simulink model "Nanogrid"  (R2026a)
settings: Solver=VariableStepAuto  StopTime=3
PreLoadFcn:
  | NanogridParam
undefined symbols (not defined in the file): baseLoad, bessSystem, bessVoltage, DiscIntNeverNeededParam, ee_sli_rtmsupport, gcbh, gflInverter, gfmInverter, nanoLoad, PV, PVInverter, ref, solar, solarInsolationChange, Ts
libraries: nesl_utility x51, eeGeneralControl x38, ee_lib x33, fl_lib x24, simulink x20, eeTransforms x13, slpidlib x8, nesl_utility_internal x4, sl_signal_attributes x4, sl_discontinuities x4, eeSinusoidalMeasurementV2 x3, batteryecm_lib x2
(part 3 of 6)

== system Nanogrid/BESS Integrated/Detailed/BESS Controller/Grid Forming ==
  VRef : Inport
  FRef : Inport  Port=2
  PRef : Inport  Port=3
  QRef : Inport  Port=4
  Mode : Inport  Port=5
  Reset : Inport  Port=6
  Bus Element In : Inport  Port=7  PortName=VIBus  Element=Vabc
  BusElementIn : Inport  Port=7  PortName=VIBus  Element=Iabc
  Current Limiting : Subsystem
  Grid Voltage Reactive Power Support : Subsystem
  Measurement : Subsystem
      mask Display: image('meas2_1_7_7_2.png');
  Power Control : Subsystem
  Subsystem2 : Subsystem
      settings: PortSchema="{\"entries\":[{\"content\":{\"sides\":[{\"content\":{\"connectorIds\":[\"Out1\"]},\"type\":\"ConnectorPlacement.EquallySpacedRectSide\",\"uuid\":\"7526c1f7-0aba-4355-8bbd-47d168879ecb\"},{\"content\":{\"connectorIds\":[\"In1\",\"In2\"],\"side\":\"RIGHT\"},\"type\":\"ConnectorPlacement.EquallySpacedRectSide\",\"uuid\":\"1dda9693-ec76-4df0-8ad4-aaa83d2574b3\"},{\"content\":{\"side\":\"TOP\"},\"type\":\"ConnectorPlacement.EquallySpacedRectSide\",\"uuid\":\"71ea411b-eb5f-4279-ae23-08ebb3ff1ed6\"}]},\"type\":\"ConnectorPlacement.EquallySpacedConnector\",\"uuid\":\"19864e0c-0998-460d-9705-13c69283d4ec\"}],\"packageUris\":[\"http://schema.mathworks.com/mf0/Connector/R2020b\"],\"version\":\"1.0\"}"
  Terminator : Terminator
  Terminator1 : Terminator
  Terminator2 : Terminator
  VoltageCurrentControl : Subsystem
      settings: PortSchema="{\"entries\":[{\"content\":{\"sides\":[{\"content\":{\"connectorIds\":[\"In1\",\"In2\",\"In3\"]},\"type\":\"ConnectorPlacement.EquallySpacedRectSide\",\"uuid\":\"0bf15a12-7bc0-47e4-89bd-435769673763\"},{\"content\":{\"connectorIds\":[\"Out1\"],\"side\":\"RIGHT\"},\"type\":\"ConnectorPlacement.EquallySpacedRectSide\",\"uuid\":\"44a15d74-8878-4ec6-abe4-be0b1b609519\"},{\"content\":{\"connectorIds\":[\"In4\"],\"side\":\"TOP\"},\"type\":\"ConnectorPlacement.EquallySpacedRectSide\",\"uuid\":\"7a96781e-5638-4b2a-8101-d5785aae9f0f\"}]},\"type\":\"ConnectorPlacement.EquallySpacedConnector\",\"uuid\":\"4b3373ad-cf20-4175-894e-3bd1604dd0ce\"}],\"packageUris\":[\"http://schema.mathworks.com/mf0/Connector/R2020b\"],\"version\":\"1.0\"}"
  mabc : Outport
  wires:
  Reset/1 -> Subsystem2/2(Reset), VoltageCurrentControl/3(Reset)
  Mode/1 -> Power Control/6(CntrlFlag)
  VRef/1 -> Power Control/4(Vref)
  FRef/1 -> Power Control/5(Fref)
  Measurement/4(fmeas) -> Terminator2/1
  Grid Voltage Reactive Power Support/2(Qref) -> Power Control/3(Qref)
  Grid Voltage Reactive Power Support/1(Pref) -> Power Control/2(Pref)
  PRef/1 -> Grid Voltage Reactive Power Support/2(PrefInput)
  QRef/1 -> Grid Voltage Reactive Power Support/3(QrefInput)
  Current Limiting/1(currentLimiting) -> VoltageCurrentControl/1(currentLimiting)
  Power Control/2(activeControl) -> VoltageCurrentControl/2(activeControl)
  Power Control/1(reactiveControl) -> Current Limiting/2(reactiveControl)
  Power Control/3(angle) -> Measurement/3(Angle)
  Measurement/1(measure) -> Grid Voltage Reactive Power Support/1(measure), Power Control/1(measure), VoltageCurrentControl/4(measure), Current Limiting/1(measure)
  Measurement/3(Qmeas) -> Terminator1/1
  Measurement/2(Pmeas) -> Terminator/1
  BusElementIn/1 -> Measurement/2(Igabc)
  Bus Element In/1 -> Measurement/1(Vgabcc)
  VoltageCurrentControl/1(mabc) -> Subsystem2/1(In)
  Subsystem2/1(mabc) -> mabc/1

== system Nanogrid/BESS Integrated/Detailed/BESS Plant/Converter ==
  mabc : Inport
  Average : Subsystem  VariantControl=Average
  Switching : Subsystem  VariantControl=Switching
  + : PMIOPort  Side=Left
  - : PMIOPort  Port=2  Side=Left
  ~ : PMIOPort  Port=3  Side=Right

== system Nanogrid/BESS Integrated/Detailed/Filter & Measurements/PLL & Measurements ==
  V : Inport
  I : Inport  Port=2
  Measurement1 : Subsystem
  Measurement2 : Subsystem
  Subsystem : Subsystem
  Out Bus Element : Outport  PortName=VIbus  Element=Vq
  Out Bus Element1 : Outport  PortName=VIbus  Element=Vd
  Out Bus Element2 : Outport  PortName=VIbus  Element=Freq
  Out Bus Element3 : Outport  PortName=VIbus  Element=Theta
  Out Bus Element4 : Outport  PortName=VIbus  Element=Vmag
  Out Bus Element5 : Outport  PortName=VIbus  Element=Iq
  Out Bus Element6 : Outport  PortName=VIbus  Element=Id
  Out Bus Element7 : Outport  PortName=VIbus  Element=Iabc
  Out Bus Element8 : Outport  PortName=VIbus  Element=Vabc
  wires:
  Subsystem/6(Id1) -> Out Bus Element6/1
  Subsystem/7(Iq1) -> Out Bus Element5/1
  Measurement1/1(Vg) -> Subsystem/2(Iabc), Out Bus Element7/1
  I/1 -> Measurement1/1(u)
  Subsystem/1(mag) -> Out Bus Element4/1
  Measurement2/1(Vg) -> Subsystem/1(Vabc), Out Bus Element8/1
  Subsystem/4(Vd) -> Out Bus Element1/1
  Subsystem/3(angle) -> Out Bus Element3/1
  Subsystem/5(Vq) -> Out Bus Element/1
  Subsystem/2(freq) -> Out Bus Element2/1
  V/1 -> Measurement2/1(u)

== system Nanogrid/BESS Integrated/Simplified/Grid Following/Measurements ==
  Current and Voltage Sensor (Three-Phase)5 : ee_lib/Sensors & Transducers/Current and Voltage Sensor (Three-Phase)  vMeasurementType=ee.enum.vmeasurement.lg  outputUnit=ee.enum.unit.pu  SRated=plantRating*1000 A*V  VRated=Vac V  I_specify=off  I_priority=None  I=[0, 0, 0] A  I_nominal_specify=off  I_nominal_value=1  I_nominal_unit=A  V_specify=off  V_priority=None  V=[0, 0, 0] V  V_nominal_specify=off  V_nominal_value=1  V_nominal_unit=V
      settings: InternalSimscapePortConfiguration="{\"Bottom\":[],\"Left\":[{\"id\":\"N1\",\"label\":\"~1\",\"type\":\"foundation.electrical.three_phase\"}],\"Right\":[{\"id\":\"V_output\",\"label\":\"V\",\"type\":\"output\"},{\"id\":\"I_output\",\"label\":\"I\",\"type\":\"output\"},{\"id\":\"N2\",\"label\":\"~2\",\"type\":\"foundation.electrical.three_phase\"}],\"Top\":[]}"
  Gain1 : Gain  Gain=1/(plantRating*1000)
  Gain2 : Gain  Gain=1/(plantRating*1000)
  Low-Pass Filter (Discrete or Continuous)1 : eeGeneralControl/Low-Pass Filter (Discrete or Continuous)  K=1  T=0.1  B=inf  A=-inf  init_option=Inherited from block input  x0=0  Ts=-1
  Low-Pass Filter (Discrete or Continuous)2 : eeGeneralControl/Low-Pass Filter (Discrete or Continuous)  K=1  T=0.1  B=inf  A=-inf  init_option=Inherited from block input  x0=0  Ts=-1
  PS-Simulink Converter{,1..3} (4 alike) : nesl_utility/PS-Simulink Converter  PhysicalDomain=network_engine_domain  SubClassName=ps_output  LeftPortType=input  RightPortType=output  PseudoPeriodic=off  Frequencies=[]  VectorFormat=inherit  Unit=inherit  AffineConversion=off
  Power Sensor (Three-Phase) : ee_lib/Sensors & Transducers/Power Sensor (Three-Phase)  load_type=ee.enum.passive.type_balanced.balanced  f0=60 Hz
      settings: InternalSimscapePortConfiguration="{\"Bottom\":[],\"Left\":[{\"id\":\"N1\",\"label\":\"~1\",\"type\":\"foundation.electrical.three_phase\"}],\"Right\":[{\"id\":\"N2\",\"label\":\"~2\",\"type\":\"foundation.electrical.three_phase\"}],\"Top\":[{\"id\":\"Pm\",\"label\":\"P\",\"type\":\"output\"},{\"id\":\"Qm\",\"label\":\"Q\",\"type\":\"output\"}]}"
  In : PMIOPort  Side=Left
  ~ : PMIOPort  Port=2  Side=Right
  P : Outport
  Q : Outport  Port=2
  V : Outport  Port=3
  I : Outport  Port=4
  wires:
  Gain2/1 -> Q/1
  Gain1/1 -> P/1
  PS-Simulink Converter3/1 -> I/1
  PS-Simulink Converter2/1 -> V/1
  Low-Pass Filter (Discrete or Continuous)2/1 -> Gain2/1
  Low-Pass Filter (Discrete or Continuous)1/1 -> Gain1/1
  PS-Simulink Converter1/1 -> Low-Pass Filter (Discrete or Continuous)2/1
  PS-Simulink Converter/1 -> Low-Pass Filter (Discrete or Continuous)1/1
  connections:
  PS-Simulink Converter3/LConn1 -- Current and Voltage Sensor (Three-Phase)5/RConn2
  Power Sensor (Three-Phase)/RConn1 -- Current and Voltage Sensor (Three-Phase)5/LConn1
  PS-Simulink Converter1/LConn1 -- Power Sensor (Three-Phase)/LConn3
  ~/RConn1 -- Current and Voltage Sensor (Three-Phase)5/RConn3
  In/RConn1 -- Power Sensor (Three-Phase)/LConn1
  PS-Simulink Converter/LConn1 -- Power Sensor (Three-Phase)/LConn2
  PS-Simulink Converter2/LConn1 -- Current and Voltage Sensor (Three-Phase)5/RConn1

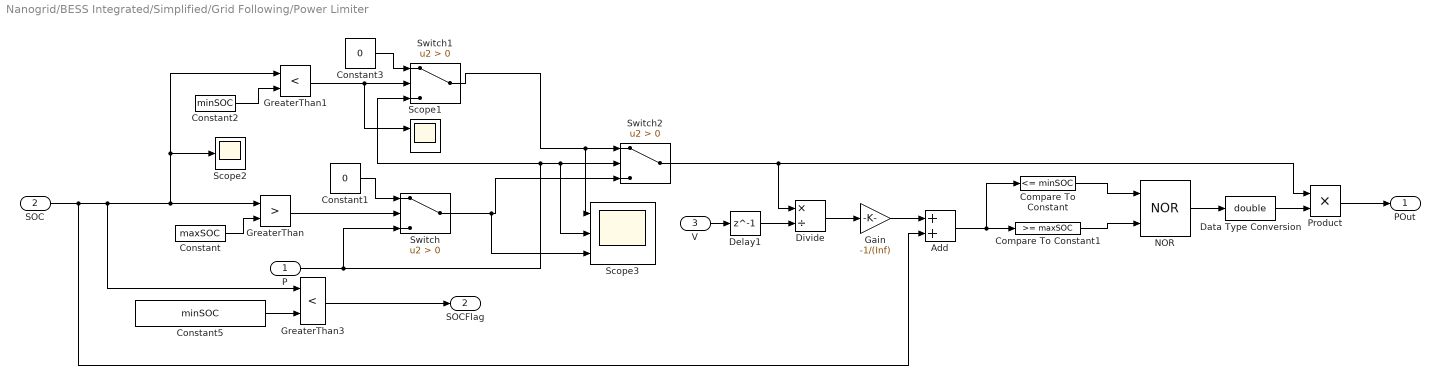
== system Nanogrid/BESS Integrated/Simplified/Grid Following/Power Limiter ==
  P : Inport
  SOC : Inport  Port=2
  V : Inport  Port=3
  Add : Sum
  Compare To Constant : simulink/Logic and Bit Operations/Compare To Constant  relop=<=  const=minSOC  OutDataTypeStr=boolean
  Compare To Constant1 : simulink/Logic and Bit Operations/Compare To Constant  relop=>=  const=maxSOC  OutDataTypeStr=boolean
  Constant : Constant  Value=maxSOC
  Constant1 : Constant  Value=0
  Constant2 : Constant  Value=minSOC
  Constant3 : Constant  Value=0
  Constant5 : Constant  Value=minSOC
  Data Type Conversion : DataTypeConversion  OutDataTypeStr=double  SaturateOnIntegerOverflow=off  RndMeth=Floor
  Delay1 : Delay  DelayLength=1
  Divide : Product  Inputs=*/
  Gain : Gain  Gain=-1/(Inf)
  GreaterThan : RelationalOperator  Operator=>  OutDataTypeStr=boolean  RndMeth=Simplest  InputSameDT=off
  GreaterThan1 : RelationalOperator  Operator=<  OutDataTypeStr=boolean  RndMeth=Simplest  InputSameDT=off
  GreaterThan3 : RelationalOperator  Operator=<  OutDataTypeStr=boolean  RndMeth=Simplest  InputSameDT=off
  NOR : Logic  Operator=NOR  IconShape=distinctive  AllPortsSameDT=off  OutDataTypeStr=boolean
  Product : Product
  Scope1 : Scope  NumInputPorts=2
  Scope2 : Scope
  Scope3 : Scope  NumInputPorts=3
  Switch : Switch  Criteria=u2 > Threshold  SaturateOnIntegerOverflow=off  InputSameDT=off
  Switch1 : Switch  Criteria=u2 > Threshold  SaturateOnIntegerOverflow=off  InputSameDT=off
  Switch2 : Switch  Criteria=u2 > Threshold  SaturateOnIntegerOverflow=off  InputSameDT=off
  POut : Outport
  SOCFlag : Outport  Port=2
  wires:
  Product/1 -> POut/1
  Gain/1 -> Add/1
  Data Type Conversion/1 -> Product/2
  NOR/1 -> Data Type Conversion/1
  Compare To Constant1/1 -> NOR/2
  Compare To Constant/1 -> NOR/1
  Add/1 -> Compare To Constant1/1, Compare To Constant/1
  Switch2/1 -> Product/1, Divide/1
  Switch/1 -> Switch2/3, Scope3/3
  SOC/1 -> GreaterThan/1, GreaterThan1/1, Scope2/1, GreaterThan3/1, Add/2
  Divide/1 -> Gain/1
  Delay1/1 -> Divide/2
  V/1 -> Delay1/1
  GreaterThan3/1 -> SOCFlag/1
  Constant5/1 -> GreaterThan3/2
  Constant/1 -> GreaterThan/2
  GreaterThan/1 -> Switch/2
  Constant1/1 -> Switch/1
  Constant2/1 -> GreaterThan1/2
  GreaterThan1/1 -> Switch1/2, Scope1/1
  Constant3/1 -> Switch1/1
  Switch1/1 -> Switch2/1, Scope3/1
  P/1 -> Switch/3, Switch1/3, Switch2/2, Scope3/2

== system Nanogrid/BESS Integrated/Simplified/Grid Following/SOC Estimation ==
  I : Inport
  Constant : Constant  Value=0.95
  Gain : Gain  Gain=-1/(100000)
  Integrator (Discrete or Continuous) : eeGeneralControl/Integrator (Discrete or Continuous)  LabelModeActiveChoice=Discrete  IntegratorMethod=Integration: Forward Euler  ExternalReset=level  LimitType=Anti-windup  B=inf  A=-inf  Ts=-1
  SOC : Outport
  wires:
  Integrator (Discrete or Continuous)/1 -> SOC/1
  Gain/1 -> Integrator (Discrete or Continuous)/1
  I/1 -> Gain/1
  Constant/1 -> Integrator (Discrete or Continuous)/3

== system Nanogrid/BESS Integrated/Simplified/Grid Forming/Limiter ==
  SOC : Inport
  Compare To Constant : simulink/Logic and Bit Operations/Compare To Constant  relop=<=  const=minSOC  OutDataTypeStr=boolean
  Compare To Constant1 : simulink/Logic and Bit Operations/Compare To Constant  relop=>=  const=maxSOC  OutDataTypeStr=boolean
  Data Type Conversion : DataTypeConversion  OutDataTypeStr=double  SaturateOnIntegerOverflow=off  RndMeth=Floor
  Delay : Delay  DelayLength=1  InputProcessing=Columns as channels (frame based)
  OR : Logic  Operator=OR  AllPortsSameDT=off  OutDataTypeStr=boolean
  Flag : Outport
  wires:
  Delay/1 -> Flag/1
  Data Type Conversion/1 -> Delay/1
  OR/1 -> Data Type Conversion/1
  Compare To Constant1/1 -> OR/2
  Compare To Constant/1 -> OR/1
  SOC/1 -> Compare To Constant1/1, Compare To Constant/1

== system Nanogrid/BESS Integrated/Simplified/Grid Forming/Measurements ==
  Current and Voltage Sensor (Three-Phase)5 : ee_lib/Sensors & Transducers/Current and Voltage Sensor (Three-Phase)  vMeasurementType=ee.enum.vmeasurement.lg  outputUnit=ee.enum.unit.pu  SRated=plantRating*1000 A*V  VRated=Vac V  I_specify=off  I_priority=None  I=[0, 0, 0] A  I_nominal_specify=off  I_nominal_value=1  I_nominal_unit=A  V_specify=off  V_priority=None  V=[0, 0, 0] V  V_nominal_specify=off  V_nominal_value=1  V_nominal_unit=V
      settings: InternalSimscapePortConfiguration="{\"Bottom\":[],\"Left\":[{\"id\":\"N1\",\"label\":\"~1\",\"type\":\"foundation.electrical.three_phase\"}],\"Right\":[{\"id\":\"V_output\",\"label\":\"V\",\"type\":\"output\"},{\"id\":\"I_output\",\"label\":\"I\",\"type\":\"output\"},{\"id\":\"N2\",\"label\":\"~2\",\"type\":\"foundation.electrical.three_phase\"}],\"Top\":[]}"
  Gain1 : Gain  Gain=1/(plantRating*1000)
  Gain2 : Gain  Gain=1/(plantRating*1000)
  PS-Simulink Converter{,1..3} (4 alike) : nesl_utility/PS-Simulink Converter  PhysicalDomain=network_engine_domain  SubClassName=ps_output  LeftPortType=input  RightPortType=output  PseudoPeriodic=off  Frequencies=[]  VectorFormat=inherit  Unit=inherit  AffineConversion=off
  Power Sensor (Three-Phase) : ee_lib/Sensors & Transducers/Power Sensor (Three-Phase)  load_type=ee.enum.passive.type_balanced.balanced  f0=60 Hz
      settings: InternalSimscapePortConfiguration="{\"Bottom\":[],\"Left\":[{\"id\":\"N1\",\"label\":\"~1\",\"type\":\"foundation.electrical.three_phase\"}],\"Right\":[{\"id\":\"N2\",\"label\":\"~2\",\"type\":\"foundation.electrical.three_phase\"}],\"Top\":[{\"id\":\"Pm\",\"label\":\"P\",\"type\":\"output\"},{\"id\":\"Qm\",\"label\":\"Q\",\"type\":\"output\"}]}"
  In : PMIOPort  Side=Left
  ~ : PMIOPort  Port=2  Side=Right
  P : Outport
  Q : Outport  Port=2
  V : Outport  Port=3
  I : Outport  Port=4
  wires:
  PS-Simulink Converter1/1 -> Gain2/1
  PS-Simulink Converter/1 -> Gain1/1
  PS-Simulink Converter2/1 -> V/1
  PS-Simulink Converter3/1 -> I/1
  Gain1/1 -> P/1
  Gain2/1 -> Q/1
  connections:
  PS-Simulink Converter2/LConn1 -- Current and Voltage Sensor (Three-Phase)5/RConn1
  PS-Simulink Converter/LConn1 -- Power Sensor (Three-Phase)/LConn2
  In/RConn1 -- Power Sensor (Three-Phase)/LConn1
  ~/RConn1 -- Current and Voltage Sensor (Three-Phase)5/RConn3
  PS-Simulink Converter1/LConn1 -- Power Sensor (Three-Phase)/LConn3
  Power Sensor (Three-Phase)/RConn1 -- Current and Voltage Sensor (Three-Phase)5/LConn1
  PS-Simulink Converter3/LConn1 -- Current and Voltage Sensor (Three-Phase)5/RConn2

== system Nanogrid/BESS Integrated/Simplified/Grid Forming/Reference Generator ==
  Mode : Inport
  PRef : Inport  Port=2
  P : Inport  Port=3
  QRef : Inport  Port=4
  Q : Inport  Port=5
  VRef : Inport  Port=6
  V : Inport  Port=7
  Gain : Gain  Gain=efficiency/100
  Gain2 : Gain  Gain=sqrt(3)/Vac
  If : If
  If Action Subsystem : Subsystem  TreatAsAtomicUnit=on
  If Action Subsystem1 : Subsystem  TreatAsAtomicUnit=on
  Merge : Merge
  Merge1 : Merge
  Vt : Outport
  Ph : Outport  Port=2
  wires:
  Gain/1 -> If Action Subsystem/1(PRef)
  Mode/1 -> If/1
  If/1 -> If Action Subsystem/Action
  PRef/1 -> Gain/1, If Action Subsystem1/1(PRef)
  QRef/1 -> If Action Subsystem/3(QRef)
  VRef/1 -> If Action Subsystem1/3(VRef)
  V/1 -> Gain2/1
  If/2 -> If Action Subsystem1/Action
  If Action Subsystem/1(Vt) -> Merge/1
  If Action Subsystem1/1(Vt) -> Merge/2
  If Action Subsystem/2(Ph) -> Merge1/1
  If Action Subsystem1/2(Ph) -> Merge1/2
  Merge1/1 -> Ph/1
  P/1 -> If Action Subsystem/2(P), If Action Subsystem1/2(P)
  Q/1 -> If Action Subsystem/4(Q)
  Gain2/1 -> If Action Subsystem1/4(V)
  Merge/1 -> Vt/1

== system Nanogrid/BESS Integrated/Simplified/Grid Forming/SOC Estimation ==
  P : Inport
  Constant : Constant  Value=Vdc
  Constant1 : Constant  Value=initialSOC
  Constant2 : Constant  Value=capacity
  Constant3 : Constant  Value=Inf
  Divide : Product  Inputs=*/
  Divide1 : Product  Inputs=*/
  Gain : Gain  Gain=-plantRating*1000
  Integrator (Discrete or Continuous) : eeGeneralControl/Integrator (Discrete or Continuous)  LabelModeActiveChoice=Discrete  IntegratorMethod=Integration: Forward Euler  ExternalReset=level  LimitType=Anti-windup  B=inf  A=-inf  Ts=-1
  String Compare : StringCompare
  String Constant : StringConstant  String=capacityType
  String Constant1 : StringConstant  String="\"Fixed\""
  Switch : Switch  Criteria=u2 > Threshold  SaturateOnIntegerOverflow=off  InputSameDT=off
  Meas : Outport
  wires:
  Gain/1 -> Divide/1
  P/1 -> Gain/1
  Constant/1 -> Divide/2
  Divide/1 -> Divide1/1
  Constant1/1 -> Integrator (Discrete or Continuous)/3
  Integrator (Discrete or Continuous)/1 -> Meas/1
  String Constant/1 -> String Compare/1
  String Constant1/1 -> String Compare/2
  String Compare/1 -> Switch/2
  Switch/1 -> Divide1/2
  Divide1/1 -> Integrator (Discrete or Continuous)/1
  Constant2/1 -> Switch/1
  Constant3/1 -> Switch/3

== system Nanogrid/Solar Plant Integrated/Detailed/PV Plant & Controller/Controller ==
  Qref : Inport
  ipv (A) : Inport  Port=2
  vdc (V) : Inport  Port=3
  Vabc : Inport  Port=4
  Iabc : Inport  Port=5
  Pref : Inport  Port=6
  Mode : Inport  Port=7
  If : If
  MPPT : Subsystem  TreatAsAtomicUnit=on
  Merge : Merge
  Power Reference : Subsystem  TreatAsAtomicUnit=on
  vabcRef (pu) : Outport
  wires:
  ipv (A)/1 -> MPPT/2(ipv (A))
  vdc (V)/1 -> MPPT/3(vdc (V))
  Qref/1 -> MPPT/1(Qref), Power Reference/4(QRef)
  Iabc/1 -> Power Reference/1(Iabc), MPPT/5(Iabc)
  Pref/1 -> Power Reference/3(PRef)
  Vabc/1 -> Power Reference/2(Vabc), MPPT/4(Vabc)
  If/1 -> MPPT/Action
  If/2 -> Power Reference/Action
  MPPT/1(mabc) -> Merge/1
  Power Reference/1(mabc) -> Merge/2
  Merge/1 -> vabcRef (pu)/1
  Mode/1 -> If/1

== system Nanogrid/Solar Plant Integrated/Detailed/PV Plant & Controller/PV Plant ==
  mabc : Inport
  Converter : Subsystem  InitFcn=%solar.mask.restoreConverterLink(gcb);  Variant=on  VariantControlMode=label  LabelModeActiveChoice=Average  mask{converterFidelity=Average, fSw=fSw}
      mask prompts: converterFidelity "Converter Fidelity"; fSw "Switching Frequency (kHz)"
      settings: PreSaveFcn=%solar.mask.restoreConverterLink  CloseFcn=%solar.mask.restoreConverterLink
      mask TypeOptions converterFidelity: Average | Switching
      mask Callback converterFidelity: component.mask.converterFidelity(gcb);
      mask DialogControl editSwitch Prompt: Edit converter parameters
      mask DialogControl editSwitch Callback:
      | converterFidelity = get_param(gcb,'converterFidelity');
      | blockPath = [gcb,'/',converterFidelity,'/','Converter'];
      | component.mask.openBlock(blockPath);
  Current Sensor : fl_lib/Electrical/Electrical Sensors/Current Sensor
  DC- Capacitor : fl_lib/Electrical/Electrical Elements/Capacitor  c=capDC F  r=1e-6 Ohm  g=0 1/Ohm  i_specify=off  i_priority=None  i=0 A  i_nominal_specify=off  i_nominal_value=1  i_nominal_unit=A  v_specify=off  v_priority=None  v=6560*.5 V  v_nominal_specify=off  v_nominal_value=1  v_nominal_unit=V  vc_specify=on  vc_priority=None  vc=ceil(Vac*sqrt(2)*1.2) V  vc_nominal_specify=off  vc_nominal_value=1  vc_nominal_unit=V
  ERef1 : fl_lib/Electrical/Electrical Elements/Electrical Reference
  PS-Simulink Converter : nesl_utility/PS-Simulink Converter  PhysicalDomain=network_engine_domain  SubClassName=ps_output  LeftPortType=input  RightPortType=output  PseudoPeriodic=off  Frequencies=[]  VectorFormat=inherit  Unit=inherit  AffineConversion=off
  PS-Simulink Converter1 : nesl_utility/PS-Simulink Converter  PhysicalDomain=network_engine_domain  SubClassName=ps_output  LeftPortType=input  RightPortType=output  PseudoPeriodic=off  Frequencies=[]  VectorFormat=inherit  Unit=inherit  AffineConversion=off
  PV Array : ee_lib/Sources/Solar Cell  PartSpecification="{\"CollectionId\":\"SimscapeElectrical\",\"DatasetId\":\"Tata_Power_Solar|TP300|simscape.electrical.solarCell\",\"DisplayName\":\"Tata_Power_Solar:TP300\"}"  prm=ee.enum.sources.solar_cell_prm.fiveParameter  Isc=8.71 % Datasheet derived A  Voc=0.62223 % Datasheet derived V  Is=1.08146075786774e-06 % Datasheet derived A  Is2=5.42602984007438e-09 % Datasheet derived A  Iph=8.71000410148422 % Datasheet derived A  Ir0=1000 % Datasheet derived W/m^2  ec=1.52301308864556 % Datasheet derived  N2=1.87068753668451 % Datasheet derived  Rs=0.000339119125335165 % Datasheet derived Ohm  Rp=655.536158839936 % Datasheet derived Ohm  N_series=72*nSeries% Datasheet derived  N_parallel=1*nParallel % Datasheet derived  TIPH1=0.000579985599628516 % Datasheet derived 1/K  EG=1.12 % Datasheet derived eV  TXIS1=3.78147935095899 % Datasheet derived  TXIS2=12.1162776751811 % Datasheet derived  TRS1=0.141899818875295 % Datasheet derived  TRP1=0 % Parameter not set  Tmeas=25 % Datasheet derived degC  TFIXED=25 % Datasheet derived degC  thermal_mass=100 % Parameter not set J/K  initial_temperature=25 degC
      settings: AttributesFormatString=Tata_Power_Solar:TP300
  Voltage Sensor : fl_lib/Electrical/Electrical Sensors/Voltage Sensor
  ABC : PMIOPort  Side=Right
  Ir : PMIOPort  Port=2  Side=Left
  I : Outport
  V : Outport  Port=2
  wires:
  PS-Simulink Converter/1 -> I/1
  PS-Simulink Converter1/1 -> V/1
  mabc/1 -> Converter/1(mabc)
  connections:
  PV Array/LConn2 -- Current Sensor/LConn1
  ABC/RConn1 -- Converter/RConn1
  Ir/RConn1 -- PV Array/LConn1
  PS-Simulink Converter/LConn1 -- Current Sensor/RConn1
  PS-Simulink Converter1/LConn1 -- Voltage Sensor/RConn1
  DC- Capacitor/LConn1 -- Converter/LConn1 -- Current Sensor/RConn2 -- Voltage Sensor/LConn1
  DC- Capacitor/RConn1 -- Converter/LConn2 -- ERef1/LConn1 -- PV Array/RConn1 -- Voltage Sensor/RConn2

== system Nanogrid/Solar Plant Integrated/Detailed/PV Plant & Controller/Sensor Dynamics ==
  Iin : Inport
  Vin : Inport  Port=2
  Current Measurement : Subsystem
  Product : Product
  Scope : Scope
      settings: ActiveDisplayYMinimum=-1.17977100562E+6  ActiveDisplayYMaximum=5.50264896669E+6  DataLoggingVariableName=ScopeData5
  Voltage Measurement : Subsystem
  I : Outport
  V : Outport  Port=2
  wires:
  Current Measurement/1(V) -> Product/2, I/1
  Iin/1 -> Current Measurement/1(u)
  Vin/1 -> Voltage Measurement/1(u)
  Voltage Measurement/1(I) -> Product/1, V/1
  Product/1 -> Scope/1

== system Nanogrid/BESS Integrated/Detailed/BESS Controller/Grid Following/Current_controller ==
  id-ref : Inport
  ipvd : Inport  Port=2
  iqref : Inport  Port=3
  iq : Inport  Port=4
  Vd : Inport  Port=5
  Vq : Inport  Port=6
  Constant4 : Constant  Value=0
  Gain1 : Gain  Gain=2*1*pi*frequency*L/zbase
  Gain2 : Gain  Gain=2*1*pi*frequency*L/zbase
  Mux1 : Mux  Inputs=3
  PID Controller : slpidlib/PID Controller  Controller=PID  Form=Parallel  TimeDomain=Discrete-time  UseExternalTs=off  SampleTime=-1  IntegratorMethod=Forward Euler  FilterMethod=Forward Euler  ControllerParametersSource=internal  P=Kpic  I=Kiic  UseKiTs=off  D=Kd  UseExternalDerivativeSource=off  N=100  UseFilter=on  TunerSelectOption=Transfer Function Based (PID Tuner App)  InitialConditionSource=internal  InitialConditionForIntegrator=0  InitialConditionForFilter=0  DifferentiatorICPrevScaledInput=0  ExternalReset=none  TrackingMode=off  Kt=1  LimitOutput=off  SatLimitsSource=internal  UpperSaturationLimit=inf  LowerSaturationLimit=-inf  LinearizeAsGain=on  AntiWindupMode=none  Kb=1  LimitIntegrator=off  UpperIntegratorSaturationLimit=inf  LowerIntegratorSaturationLimit=-inf  POutMin=[]  POutMax=[]  IOutMin=[]  IOutMax=[]  DOutMin=[]  DOutMax=[]  NOutMin=[]  NOutMax=[]  SumOutMin=[]  SumOutMax=[]  SaturationOutMin=[]  SaturationOutMax=[]  PParamMin=[]  PParamMax=[]  IParamMin=[]  IParamMax=[]  DParamMin=[]  DParamMax=[]  NParamMin=[]  NParamMax=[]  KbParamMin=[]  KbParamMax=[]  KtParamMin=[]  KtParamMax=[]  KbOutMin=[]  KbOutMax=[]  KtOutMin=[]  KtOutMax=[]  IntegratorOutMin=[]  IntegratorOutMax=[]  FilterOutMin=[]  FilterOutMax=[]  SumI1OutMin=[]  SumI1OutMax=[]  SumI2OutMin=[]  SumI2OutMax=[]  SumI3OutMin=[]  SumI3OutMax=[]  SumI4OutMin=[]  SumI4OutMax=[]  SumDOutMin=[]  SumDOutMax=[]  DifferentiatorOutMin=[]  DifferentiatorOutMax=[]  FilterDiffOutCoefMin=[]  FilterDiffOutCoefMax=[]  ReciprocalOutMin=[]  ReciprocalOutMax=[]  SumDenOutMin=[]  SumDenOutMax=[]  SumNumOutMin=[]  SumNumOutMax=[]  DivideOutMin=[]  DivideOutMax=[]  UdiffTsProdOutMin=[]  UdiffTsProdOutMax=[]  NTsProdOutMin=[]  NTsProdOutMax=[]  UintegralTsProdOutMin=[]  UintegralTsProdOutMax=[]  UngainTsProdOutMin=[]  UngainTsProdOutMax=[]  ClampingZeroOutDataTypeStr=Inherit: Inherit via back propagation  ClampingZeroOutMin=[]  ClampingZeroOutMax=[]  FilterDenConstantOutDataTypeStr=Inherit: Inherit via back propagation  FilterDenConstantOutMin=[]  FilterDenConstantOutMax=[]  PCopyOutDataTypeStr=Inherit: Inherit via back propagation  PCopyOutMin=[]  PCopyOutMax=[]  NCopyOutDataTypeStr=Inherit: Inherit via back propagation  NCopyOutMin=[]  NCopyOutMax=[]  IntegratorContinuousStateAttributes=''  IntegratorStateMustResolveToSignalObject=off  IntegratorRTWStateStorageClass=Auto  FilterContinuousStateAttributes=''  FilterStateMustResolveToSignalObject=off  FilterRTWStateStorageClass=Auto  ParallelPVariant=InternalParameters  IdealPVariant=Disabled  IVariant=InternalParameters  DVariant=InternalParameters  IntegratorVariant=Discrete  SatVariant=Disabled  AWVariant=Passthrough  PCopyVariant=Disabled  TRVariant=Disabled  FdbkBlocksVariant=Forward  IdealPFdbkVariant=Disabled  SatFdbkVariant=Disabled  DerivativeFilterVariant=ForwardEulerFilter  NVariant=InternalParameters  NCopyVariant=Disabled  FilterICVariant=InternalICsFilter  IntegratorICVariant=InternalICs  ExternalResetVariant=Disabled  TRSumVariant=Passthrough  SumFdbkVariant=Disabled  SumVariant=Sum_PID  TsampFilterVariant=InternalTs  TsampNgainVariant=Passthrough  TsampIntegralVariant=Disabled_SignalSpec  ExternalSaturationOutDataTypeStr=Inherit: Same as second input  DerivativeSourceVariant=ErrorSignal  PreIntVariant=InternalPreInt
  PID Controller1 : slpidlib/PID Controller  Controller=PID  Form=Parallel  TimeDomain=Discrete-time  UseExternalTs=off  SampleTime=-1  IntegratorMethod=Forward Euler  FilterMethod=Forward Euler  ControllerParametersSource=internal  P=Kpic  I=Kiic  UseKiTs=off  D=Kd  UseExternalDerivativeSource=off  N=100  UseFilter=on  TunerSelectOption=Transfer Function Based (PID Tuner App)  InitialConditionSource=internal  InitialConditionForIntegrator=0  InitialConditionForFilter=0  DifferentiatorICPrevScaledInput=0  ExternalReset=none  TrackingMode=off  Kt=1  LimitOutput=off  SatLimitsSource=internal  UpperSaturationLimit=inf  LowerSaturationLimit=-inf  LinearizeAsGain=on  AntiWindupMode=none  Kb=1  LimitIntegrator=off  UpperIntegratorSaturationLimit=inf  LowerIntegratorSaturationLimit=-inf  POutMin=[]  POutMax=[]  IOutMin=[]  IOutMax=[]  DOutMin=[]  DOutMax=[]  NOutMin=[]  NOutMax=[]  SumOutMin=[]  SumOutMax=[]  SaturationOutMin=[]  SaturationOutMax=[]  PParamMin=[]  PParamMax=[]  IParamMin=[]  IParamMax=[]  DParamMin=[]  DParamMax=[]  NParamMin=[]  NParamMax=[]  KbParamMin=[]  KbParamMax=[]  KtParamMin=[]  KtParamMax=[]  KbOutMin=[]  KbOutMax=[]  KtOutMin=[]  KtOutMax=[]  IntegratorOutMin=[]  IntegratorOutMax=[]  FilterOutMin=[]  FilterOutMax=[]  SumI1OutMin=[]  SumI1OutMax=[]  SumI2OutMin=[]  SumI2OutMax=[]  SumI3OutMin=[]  SumI3OutMax=[]  SumI4OutMin=[]  SumI4OutMax=[]  SumDOutMin=[]  SumDOutMax=[]  DifferentiatorOutMin=[]  DifferentiatorOutMax=[]  FilterDiffOutCoefMin=[]  FilterDiffOutCoefMax=[]  ReciprocalOutMin=[]  ReciprocalOutMax=[]  SumDenOutMin=[]  SumDenOutMax=[]  SumNumOutMin=[]  SumNumOutMax=[]  DivideOutMin=[]  DivideOutMax=[]  UdiffTsProdOutMin=[]  UdiffTsProdOutMax=[]  NTsProdOutMin=[]  NTsProdOutMax=[]  UintegralTsProdOutMin=[]  UintegralTsProdOutMax=[]  UngainTsProdOutMin=[]  UngainTsProdOutMax=[]  ClampingZeroOutDataTypeStr=Inherit: Inherit via back propagation  ClampingZeroOutMin=[]  ClampingZeroOutMax=[]  FilterDenConstantOutDataTypeStr=Inherit: Inherit via back propagation  FilterDenConstantOutMin=[]  FilterDenConstantOutMax=[]  PCopyOutDataTypeStr=Inherit: Inherit via back propagation  PCopyOutMin=[]  PCopyOutMax=[]  NCopyOutDataTypeStr=Inherit: Inherit via back propagation  NCopyOutMin=[]  NCopyOutMax=[]  IntegratorContinuousStateAttributes=''  IntegratorStateMustResolveToSignalObject=off  IntegratorRTWStateStorageClass=Auto  FilterContinuousStateAttributes=''  FilterStateMustResolveToSignalObject=off  FilterRTWStateStorageClass=Auto  ParallelPVariant=InternalParameters  IdealPVariant=Disabled  IVariant=InternalParameters  DVariant=InternalParameters  IntegratorVariant=Discrete  SatVariant=Disabled  AWVariant=Passthrough  PCopyVariant=Disabled  TRVariant=Disabled  FdbkBlocksVariant=Forward  IdealPFdbkVariant=Disabled  SatFdbkVariant=Disabled  DerivativeFilterVariant=ForwardEulerFilter  NVariant=InternalParameters  NCopyVariant=Disabled  FilterICVariant=InternalICsFilter  IntegratorICVariant=InternalICs  ExternalResetVariant=Disabled  TRSumVariant=Passthrough  SumFdbkVariant=Disabled  SumVariant=Sum_PID  TsampFilterVariant=InternalTs  TsampNgainVariant=Passthrough  TsampIntegralVariant=Disabled_SignalSpec  ExternalSaturationOutDataTypeStr=Inherit: Same as second input  DerivativeSourceVariant=ErrorSignal  PreIntVariant=InternalPreInt
  Scope : Scope  NumInputPorts=2
      settings: ActiveDisplayYMinimum=-1  ActiveDisplayYMaximum=1
  Scope1 : Scope  NumInputPorts=2
      settings: ActiveDisplayYMinimum=-1.21282  ActiveDisplayYMaximum=0.9154  DataLoggingVariableName=ScopeData2
  Sum1 : Sum  Inputs=|+-
  Sum3 : Sum  Inputs=|++-
  Sum4 : Sum  Inputs=|+++
  Sum5 : Sum  Inputs=|+-
  mdq0 : Outport
  wires:
  iqref/1 -> Sum5/1, Scope1/1
  Mux1/1 -> mdq0/1
  Sum4/1 -> [Eq], Mux1/2
  PID Controller1/1 -> Sum4/1
  Sum5/1 -> PID Controller1/1
  Constant4/1 -> Mux1/3
  Vd/1 -> Sum3/1
  Sum1/1 -> PID Controller/1
  iq/1 -> Sum5/2, Gain2/1, Scope1/2
  Vq/1 -> Sum4/2
  Gain1/1 -> Sum4/3
  id-ref/1 -> Sum1/1, Scope/1
  ipvd/1 -> Sum1/2, Gain1/1, Scope/2
  Gain2/1 -> Sum3/3
  Sum3/1 -> [Ed], Mux1/1
  PID Controller/1 -> Sum3/2

== system Nanogrid/BESS Integrated/Detailed/BESS Controller/Grid Following/Reference Current ==
  note: Avoid division by zero during start
  note: Current Limiters
  V_ref : Inport
  V-mag : Inport  Port=2
  del f : Inport  Port=3
  LVRT_iq : Inport  Port=4
  PRef : Inport  Port=5
  QRef : Inport  Port=6
  Constant1 : Constant
  Constant3 : Constant  Value=Imax
  Current limits : Subsystem
  Refernce id generation : Subsystem
  Refernce iq generation : Subsystem
  Switch : Switch  Criteria=u2 ~= 0  SaturateOnIntegerOverflow=off  InputSameDT=off
  Unit Delay1 : UnitDelay  SampleTime=Ts
  Unit Delay3 : UnitDelay  SampleTime=Ts
  id_ref : Outport
  iq_ref : Outport  Port=2
  wires:
  Current limits/2(iubd) -> Refernce id generation/3(ubid)
  PRef/1 -> Refernce id generation/4(PRef)
  QRef/1 -> Refernce iq generation/5(Q_ref)
  Constant1/1 -> Switch/3
  Switch/1 -> Refernce iq generation/3(V_mag), Refernce id generation/1(V_mag)
  V-mag/1 -> Switch/2, Switch/1
  LVRT_iq/1 -> Refernce iq generation/4(LVRT_iq)
  Refernce iq generation/1(iq_ref) -> iq_ref/1, Unit Delay1/1
  V_ref/1 -> Refernce iq generation/2(V_ref)
  del f/1 -> Refernce id generation/2(del f)
  Refernce id generation/1(id_ref) -> Unit Delay3/1, id_ref/1
  Constant3/1 -> Current limits/1(Imax)
  Unit Delay3/1 -> Current limits/3(idref)
  Current limits/1(iubq) -> Refernce iq generation/1(ubiq)
  Unit Delay1/1 -> Current limits/2(iqref)

== system Nanogrid/BESS Integrated/Detailed/BESS Controller/Grid Forming/Current Limiting ==
  In Bus Element : Inport  PortName=measure  Element=Igd
  In Bus Element1 : Inport  PortName=measure  Element=Igq
  In Bus Element2 : Inport  Port=2  PortName=reactiveControl  Element=Vmd
  In Bus Element4 : Inport  Port=2  PortName=reactiveControl  Element=Vmq
  CurrentLimitingMethod : Subsystem  Variant=on  VariantControlMode=label  VariantControl=Choice  LabelModeActiveChoice=ctSat
  Scope : Scope  NumInputPorts=2
      settings: ActiveDisplayYMinimum=-1  ActiveDisplayYMaximum=1
  Subtract : Sum  Inputs=+-
  Subtract1 : Sum  Inputs=-+
  Out Bus Element : Outport  PortName=currentLimiting  Element=Vmd
  Out Bus Element1 : Outport  PortName=currentLimiting  Element=Vmq
  Out Bus Element2 : Outport  PortName=currentLimiting  Element=Idmax
  Out Bus Element3 : Outport  PortName=currentLimiting  Element=Iqmax
  wires:
  CurrentLimitingMethod/2(delVq) -> Subtract1/1
  CurrentLimitingMethod/1(delVd) -> Subtract/2
  CurrentLimitingMethod/3(Idmax) -> Out Bus Element2/1
  In Bus Element/1 -> CurrentLimitingMethod/1(Igd)  "Q"
  CurrentLimitingMethod/4(Iqmax) -> Out Bus Element3/1
  Subtract1/1 -> Out Bus Element1/1, Scope/2
  Subtract/1 -> Out Bus Element/1, Scope/1
  In Bus Element4/1 -> Subtract1/2
  In Bus Element1/1 -> CurrentLimitingMethod/2(Igq)
  In Bus Element2/1 -> Subtract/1

== system Nanogrid/BESS Integrated/Detailed/BESS Controller/Grid Forming/Grid Voltage Reactive Power Support ==
  In Bus Element1 : Inport  PortName=measure  Element=Vgd
  In Bus Element3 : Inport  PortName=measure  Element=Vgq
  In Bus Element2 : Inport  PortName=measure  Element=Igd
  In Bus Element4 : Inport  PortName=measure  Element=Igq
  PrefInput : Inport  Port=2
  QrefInput : Inport  Port=3
  Modifying Active Power Reference : Subsystem
  Modifying Reactive Power Reference : Subsystem
  Scope : Scope
  Scope1 : Scope
      settings: ActiveDisplayYMinimum=-1  ActiveDisplayYMaximum=1
  Scope2 : Scope
      settings: ActiveDisplayYMinimum=-1  ActiveDisplayYMaximum=1
  Pref : Outport
  Qref : Outport  Port=2
  wires:
  Modifying Reactive Power Reference/2(QrefNew) -> Qref/1, Scope2/1
  Modifying Reactive Power Reference/1(PrefNew) -> Pref/1, Scope1/1
  QrefInput/1 -> Modifying Reactive Power Reference/3(Qref)
  In Bus Element3/1 -> Modifying Reactive Power Reference/2(Vgq)
  In Bus Element1/1 -> Modifying Active Power Reference/2(Vd), Modifying Reactive Power Reference/1(Vgd)
  In Bus Element4/1 -> Modifying Active Power Reference/4(Igq)
  In Bus Element2/1 -> Modifying Active Power Reference/3(Igd)
  PrefInput/1 -> Modifying Active Power Reference/1(PrefInput)
  Modifying Active Power Reference/1(Pref) -> Modifying Reactive Power Reference/4(Pref), Scope/1

== system Nanogrid/BESS Integrated/Detailed/BESS Controller/Grid Forming/Measurement ==
  Vgabcc : Inport
  Igabc : Inport  Port=2
  Angle : Inport  Port=3
  Frequency Measurement : Subsystem
  Gain1 : Gain  Gain=2/3
  Gain2 : Gain  Gain=2/3
  Gain3 : Gain  Gain=1%/(girdLineVoltage*sqrt(2/3))
  Gain4 : Gain  Gain=1%/(girdLineVoltage*sqrt(2/3))
  Gain5 : Gain  Gain=1%/(power/(sqrt(3)*girdLineVoltage)*sqrt(2))
  Gain6 : Gain  Gain=1%/(power/(sqrt(3)*girdLineVoltage)*sqrt(2))
  Power Measurement (Three-Phase) : eePowerMeasurement/Power Measurement (Three-Phase)  LabelModeActiveChoice=Discrete  F=powerFreq  K=[1]  Seq=Positive  Ts=measSampleTime
  abc2dq : Subsystem
  Out Bus Element : Outport  PortName=measure  Element=P
  Out Bus Element1 : Outport  PortName=measure  Element=Q
  Out Bus Element2 : Outport  PortName=measure  Element=Vgd
  Out Bus Element3 : Outport  PortName=measure  Element=Vgq
  Out Bus Element4 : Outport  PortName=measure  Element=Igd
  Out Bus Element5 : Outport  PortName=measure  Element=Igq
  Out Bus Element6 : Outport  PortName=measure  Element=fgrid
  Pmeas : Outport  Port=2
  Qmeas : Outport  Port=3
  fmeas : Outport  Port=4
  wires:
  Frequency Measurement/1(freq) -> fmeas/1, Out Bus Element6/1
  Gain6/1 -> Out Bus Element5/1  "Igq"
  Gain5/1 -> Out Bus Element4/1  "Igd"
  Gain4/1 -> Out Bus Element2/1  "Vgd"
  Gain3/1 -> Out Bus Element3/1  "Vgq"
  abc2dq/4(Igq) -> Gain6/1
  abc2dq/3(Igd) -> Gain5/1
  abc2dq/2(Vgq) -> Gain3/1
  abc2dq/1(Vgd) -> Gain4/1
  Gain1/1 -> Out Bus Element1/1, Qmeas/1  "Qmeas"
  Gain2/1 -> Out Bus Element/1, Pmeas/1  "Pmeas"
  Power Measurement (Three-Phase)/2 -> Gain1/1
  Igabc/1 -> Power Measurement (Three-Phase)/2, abc2dq/1(Igabc)  "Iabc"
  Power Measurement (Three-Phase)/1 -> Gain2/1
  Angle/1 -> abc2dq/2(Angle)
  Vgabcc/1 -> Power Measurement (Three-Phase)/1, Frequency Measurement/1(Vabc), abc2dq/3(Vgabc)  "Vabc"

== system Nanogrid/BESS Integrated/Detailed/BESS Controller/Grid Forming/Power Control ==
  note: Active Power Control
  note: Reactive Power Control
  In Bus Element2 : Inport  PortName=measure  Element=P
  In Bus Element1 : Inport  PortName=measure  Element=fgrid
  BusElementIn : Inport  PortName=measure  Element=Vgd
  BusElementIn2 : Inport  PortName=measure  Element=Q
  Pref : Inport  Port=2
  Qref : Inport  Port=3
  Vref : Inport  Port=4
  Fref : Inport  Port=5
  CntrlFlag : Inport  Port=6
  ActivePowerControl : Subsystem  Variant=on  VariantControlMode=label  VariantControl=Choice  LabelModeActiveChoice=vsm
  ReactiveControl : Subsystem
  Scope : Scope
      settings: ActiveDisplayYMinimum=-1  ActiveDisplayYMaximum=1  DataLoggingVariableName=ScopeData16
  Out Bus Element : Outport  PortName=reactiveControl  Element=Vmd
  Out Bus Element1 : Outport  PortName=reactiveControl  Element=Vmq
  Out Bus Element6 : Outport  Port=2  PortName=activeControl  Element=angle
  Out Bus Element4 : Outport  Port=2  PortName=activeControl  Element=w
  angle : Outport  Port=3
  wires:
  BusElementIn2/1 -> ReactiveControl/3(Qmeas)
  BusElementIn/1 -> ReactiveControl/4(Vgdmeas), Scope/1
  [Cntrlflag] -> ReactiveControl/1(CntrlFlag)
  Vref/1 -> ReactiveControl/5(Vref)
  [Cntrlflag] -> ActivePowerControl/4(cntrlflag)
  CntrlFlag/1 -> [Cntrlflag]
  Fref/1 -> ActivePowerControl/3(fref)
  In Bus Element1/1 -> ActivePowerControl/5(fgrid)
  In Bus Element2/1 -> ActivePowerControl/2(Pmeas)
  Qref/1 -> ReactiveControl/2(Qref)  "Q"
  Pref/1 -> ActivePowerControl/1(Pref)  "Q"
  ReactiveControl/2(Vmq) -> Out Bus Element1/1
  ReactiveControl/1(Vmd) -> Out Bus Element/1
  ActivePowerControl/1(Theta) -> Out Bus Element6/1, angle/1
  ActivePowerControl/2(w) -> Out Bus Element4/1

== system Nanogrid/BESS Integrated/Detailed/BESS Controller/Grid Forming/Subsystem2 ==
  In : Inport
  Reset : Inport  Port=2
  AND : Logic  IconShape=distinctive  AllPortsSameDT=off  OutDataTypeStr=boolean
  Data Type Conversion : DataTypeConversion  SaturateOnIntegerOverflow=off  RndMeth=Floor
  Delay : Delay  DelayLength=1  SampleTime=Ts*20000
  Delay1 : Delay  DelayLength=1
  NOT : Logic  Operator=NOT  IconShape=distinctive  AllPortsSameDT=off  OutDataTypeStr=boolean
  NOT1 : Logic  Operator=NOT  IconShape=distinctive  AllPortsSameDT=off  OutDataTypeStr=boolean
  Product : Product
  mabc : Outport
  wires:
  In/1 -> Product/2
  Reset/1 -> AND/1, Delay/1
  NOT/1 -> AND/2
  Delay/1 -> NOT/1
  Product/1 -> Delay1/1
  AND/1 -> NOT1/1
  NOT1/1 -> Data Type Conversion/1
  Data Type Conversion/1 -> Product/1
  Delay1/1 -> mabc/1

== system Nanogrid/BESS Integrated/Detailed/BESS Controller/Grid Forming/VoltageCurrentControl ==
  In Bus Element : Inport  PortName=currentLimiting  Element=Vmd
  In Bus Element1 : Inport  PortName=currentLimiting  Element=Vmq
  In Bus Element6 : Inport  PortName=currentLimiting  Element=Idmax
  In Bus Element7 : Inport  PortName=currentLimiting  Element=Iqmax
  Bus Element In6 : Inport  Port=2  PortName=activeControl  Element=w
  Bus Element In1 : Inport  Port=2  PortName=activeControl  Element=angle
  Reset : Inport  Port=3
  In Bus Element2 : Inport  Port=4  PortName=measure  Element=Vgd
  In Bus Element3 : Inport  Port=4  PortName=measure  Element=Vgq
  In Bus Element4 : Inport  Port=4  PortName=measure  Element=Igd
  In Bus Element5 : Inport  Port=4  PortName=measure  Element=Igq
  Controller : Subsystem
      settings: PortSchema="{\"entries\":[{\"content\":{\"sides\":[{\"content\":{\"connectorIds\":[\"In1\",\"In2\",\"In3\",\"In4\",\"In5\",\"In6\",\"In7\",\"In8\",\"In9\"]},\"type\":\"ConnectorPlacement.EquallySpacedRectSide\",\"uuid\":\"29d30ab3-0ae0-4ae6-aaee-46c6f5faca9c\"},{\"content\":{\"connectorIds\":[\"Out1\",\"Out2\"],\"side\":\"RIGHT\"},\"type\":\"ConnectorPlacement.EquallySpacedRectSide\",\"uuid\":\"4918c3a7-9f8f-4af5-ac25-a0a0710917b2\"},{\"content\":{\"connectorIds\":[\"In10\"],\"side\":\"TOP\"},\"type\":\"ConnectorPlacement.EquallySpacedRectSide\",\"uuid\":\"c6ee8000-0a39-46c2-b8e8-8b73a56a82d9\"}]},\"type\":\"ConnectorPlacement.EquallySpacedConnector\",\"uuid\":\"193e0bc8-3764-41d1-9278-3938c4a9e9f5\"}],\"packageUris\":[\"http://schema.mathworks.com/mf0/Connector/R2020b\"],\"version\":\"1.0\"}"
  Modulation Signal : Subsystem
  mabc : Outport
  wires:
  Reset/1 -> Controller/10(Reset)
  Bus Element In1/1 -> Modulation Signal/3(Angle)
  In Bus Element1/1 -> Controller/3(Vgqref)
  In Bus Element/1 -> Controller/2(Vgdref)
  Bus Element In6/1 -> Controller/1(Angfreq)
  In Bus Element3/1 -> Controller/5(Vsq)
  In Bus Element2/1 -> Controller/4(Vsd)
  In Bus Element7/1 -> Controller/9(Iqmax)
  In Bus Element6/1 -> Controller/8(Idmax)
  In Bus Element5/1 -> Controller/7(Iq)
  In Bus Element4/1 -> Controller/6(Id)
  Controller/1(Vd) -> Modulation Signal/1(Vd)
  Modulation Signal/1(mabc) -> mabc/1
  Controller/2(Vq) -> Modulation Signal/2(Vq)

== system Nanogrid/BESS Integrated/Detailed/BESS Plant/Converter/Average ==
  mabc : Inport
  Converter : ee_lib/Semiconductors & Converters/Converters/Average-Value Voltage Source Converter (Three-Phase)  port_option=ee.enum.threePhasePort.composite  enable_block_pulses_input=false  krec=0.01 Ohm  frequency_option=ee.enum.converters.frequency.variable  input_option=ee.enum.converters.inputOption.ModWave  FRated=60 Hz  losses_parameterization=ee.enum.converters.losses.fixed  Pfixed=0.5 W  ks=0.01  kc1=1.7 V  kc2=0.01 Ohm  Ploss_vect=[100, 800, 1870, 3250, 4900] W  Irms_vect=[10, 100, 200, 300, 400] A  Vdc_nom=300 V  thermal_mass=30000 J/K  temperature_specify=off  temperature_priority=High  temperature=298.15 K  temperature_nominal_specify=off  temperature_nominal_value=1  temperature_nominal_unit=K
  Simulink-PS Converter : nesl_utility/Simulink-PS Converter  PhysicalDomain=network_engine_domain  SubClassName=ps_input  LeftPortType=input  RightPortType=output  PseudoPeriodic=off  Frequencies=[]  NoiseDistribution=none  NoiseParameters=[]  Unit=1  AffineConversion=off  FilteringAndDerivatives=provide  SimscapeFilterOrder=1  InputFilterTimeConstant=0.001  UdotUserProvided=0
  + : PMIOPort  Side=Left
  - : PMIOPort  Port=2  Side=Left
  ~ : PMIOPort  Port=3  Side=Right
  wires:
  mabc/1 -> Simulink-PS Converter/1
  connections:
  Simulink-PS Converter/RConn1 -- Converter/LConn1
  ~/RConn1 -- Converter/LConn2
  -/RConn1 -- Converter/RConn2
  +/RConn1 -- Converter/RConn1

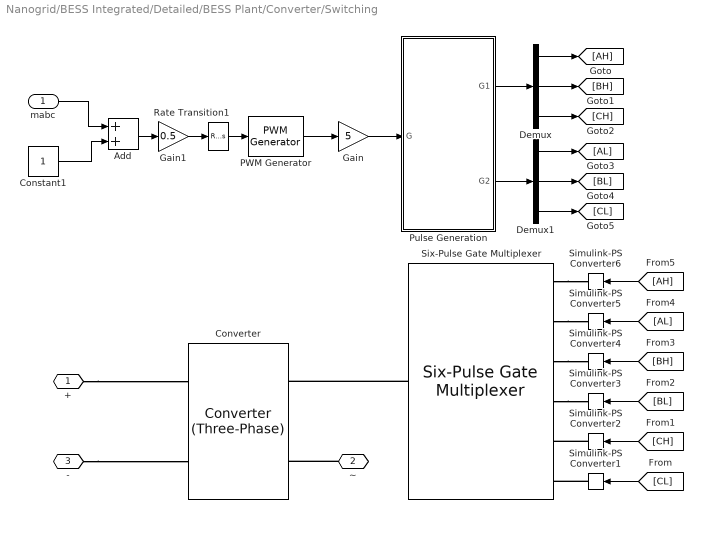
== system Nanogrid/BESS Integrated/Detailed/BESS Plant/Converter/Switching ==
  mabc : Inport
  Add : Sum
  Constant1 : Constant
  Converter : ee_lib/Semiconductors & Converters/Converters/Converter (Three-Phase)  port_option=ee.enum.threePhasePort.composite  fidelity_option=ee.enum.converters.fidelity.detailed  device_type=ee.enum.converters.switchingdevice.ideal  showThermalPort=false  K=0  Vth=1 V  Vgt=1 V  Vgt_off=-1 V  Ih=1 A  Vf=0.8 V  Ron=0.001 Ohm  Rds=0.001 Ohm  Goff=1e-6 1/Ohm  Eon_scalar=22.86e-3 J  Eoff_scalar=17.14e-3 J  Eoff_natural_commutation=10e-3 J  Voff=300 V  Iout_scalar=600 A  onCurrentMeasDelay=0 s  useCurrentFromPreviousCycle=false  useVoltageFromPreviousCycle=false  diode_param=ee.enum.converters.protectiondiode.nodynamics  diode_Vf=0.01 V  diode_Ron=0.0001 Ohm  diode_Goff=1e-5 1/Ohm  diode_C=50 nF  diode_iRM=-235 A  diode_iF=300 A  diode_idot=-50 A/us  diode_trr_param=ee.enum.converters.diodetrr.trr_factor  diode_trr_factor=3  diode_trr=15 us  diode_Qrr=1500 s*uA  diode_rec_loss_model=ee.enum.diode.reverseRecoveryModel.fixed  diode_ErecVal=0 J  diode_scaleWithIandV=false  diode_ErecMat=zeros(2, 3) J  diode_TjrecVec=[298.15, 398.15] K  diode_IfrecVec=[.1, 1, 10] A  diode_IrecVal=10 A  diode_VrecVal=10 V  diode_tFilter=1 / 1000 / 100 s  thermal_network_parameterization=ee.enum.thermalNetworkTopology.external  Rth=[.08, .5] K/W  Rth_Cauer=[.08, .1, .5] K/W  Rth_Foster=[.08, .14, .22, .16] K/W  thermal_mass_parameterization=ee.enum.thermalNetwork.timeconstant  thermal_mass=[.01, .5] J/K  thermal_mass_Cauer=[.01, .1, .5] J/K  thermal_mass_Foster=[.001, .005, .05, .5] J/K  thermal_time_constant=[.001, .2] s  thermal_time_constant_Cauer=[.001, .1, .2] s  thermal_time_constant_Foster=[7e-05, .0007, .01, .08] s  thermal_mass_initial_temperatures=[25, 25] degC  thermal_mass_initial_temperatures_Cauer=[25, 25, 25] degC  junction_thermal_mass=0.01 J/K  Tvec_initial_Foster=[25, 25, 25, 25] degC  snubber_type=ee.enum.converters.snubber.exclude  Cs=1e-7 F  Rs=0.1 Ohm  Vce_loss=[0, 150, 300] V
  Demux : Demux  Outputs=3
  Demux1 : Demux  Outputs=3
  Gain : Gain  Gain=5
  Gain1 : Gain  Gain=0.5
  PWM Generator : eePwmGenerator/PWM Generator  CarrCount=Up  Tper=1/(fSw*1000)  Tdelay=0  Ts=1/(10*fSw*1000)
  Pulse Generation : Subsystem
  Rate Transition1 : RateTransition  OutPortSampleTime=1/(10*fSw*1000)
  Simulink-PS Converter{1..6} (6 alike) : nesl_utility/Simulink-PS Converter  PhysicalDomain=network_engine_domain  SubClassName=ps_input  LeftPortType=input  RightPortType=output  PseudoPeriodic=off  Frequencies=[]  NoiseDistribution=none  NoiseParameters=[]  Unit=1  AffineConversion=off  FilteringAndDerivatives=provide  SimscapeFilterOrder=1  InputFilterTimeConstant=0.001  UdotUserProvided=0
  Six-Pulse Gate Multiplexer : ee_lib/Semiconductors & Converters/Converters/Six-Pulse Gate Multiplexer  port_option=ee.enum.controlport.ps
  + : PMIOPort  Side=Left
  ~ : PMIOPort  Port=2  Side=Right
  - : PMIOPort  Port=3  Side=Left
  wires:
  Demux1/1 -> [AL]
  [BL] -> Simulink-PS Converter3/1
  [AH] -> Simulink-PS Converter6/1
  Demux1/3 -> [CL]
  Gain1/1 -> Rate Transition1/1
  Demux/3 -> [CH]
  Demux/2 -> [BH]
  [CL] -> Simulink-PS Converter1/1
  Constant1/1 -> Add/2
  Add/1 -> Gain1/1
  Gain/1 -> Pulse Generation/1(G)
  PWM Generator/1 -> Gain/1
  mabc/1 -> Add/1
  [CH] -> Simulink-PS Converter2/1
  [AL] -> Simulink-PS Converter5/1
  Demux1/2 -> [BL]
  Demux/1 -> [AH]
  Rate Transition1/1 -> PWM Generator/1
  Pulse Generation/2(G2) -> Demux1/1
  Pulse Generation/1(G1) -> Demux/1
  [BH] -> Simulink-PS Converter4/1
  connections:
  ~/RConn1 -- Converter/LConn2
  Six-Pulse Gate Multiplexer/LConn2 -- Simulink-PS Converter5/RConn1
  Simulink-PS Converter2/RConn1 -- Six-Pulse Gate Multiplexer/LConn5
  Simulink-PS Converter1/RConn1 -- Six-Pulse Gate Multiplexer/LConn6
  Six-Pulse Gate Multiplexer/LConn3 -- Simulink-PS Converter4/RConn1
  Six-Pulse Gate Multiplexer/RConn1 -- Converter/LConn1
  Six-Pulse Gate Multiplexer/LConn1 -- Simulink-PS Converter6/RConn1
  Six-Pulse Gate Multiplexer/LConn4 -- Simulink-PS Converter3/RConn1
  +/RConn1 -- Converter/RConn1
  -/RConn1 -- Converter/RConn2

== system Nanogrid/BESS Integrated/Detailed/Filter & Measurements/PLL & Measurements/Measurement1 ==
  u : Inport
  Lead-Lag (Discrete or Continuous) : eeGeneralControl/Lead-Lag (Discrete or Continuous)  T1=0  T2=1e-3  B=inf  A=-inf  init_option=Inherited from block input  x0=0  Ts=Ts
  Vg : Outport
  wires:
  u/1 -> Lead-Lag (Discrete or Continuous)/1
  Lead-Lag (Discrete or Continuous)/1 -> Vg/1

== system Nanogrid/BESS Integrated/Detailed/Filter & Measurements/PLL & Measurements/Measurement2 ==
  u : Inport
  Lead-Lag (Discrete or Continuous) : eeGeneralControl/Lead-Lag (Discrete or Continuous)  T1=0  T2=1e-3  B=inf  A=-inf  init_option=Inherited from block input  x0=0  Ts=Ts
  Vg : Outport
  wires:
  u/1 -> Lead-Lag (Discrete or Continuous)/1
  Lead-Lag (Discrete or Continuous)/1 -> Vg/1

== system Nanogrid/BESS Integrated/Detailed/Filter & Measurements/PLL & Measurements/Subsystem ==
  Vabc : Inport
  Iabc : Inport  Port=2
  Demux : Demux  Outputs=3
  Demux1 : Demux  Outputs=3
  Park Transform : eeTransforms/Park Transform  AxisAlignment=Q-axis  PowerInvariant=off
  Park Transform1 : eeTransforms/Park Transform  AxisAlignment=Q-axis  PowerInvariant=off
  Scope : Scope  NumInputPorts=2
      settings: ActiveDisplayYMinimum=0.95416  ActiveDisplayYMaximum=1.02793  DataLoggingVariableName=ScopeData5
  Scope1 : Scope  NumInputPorts=2
      settings: ActiveDisplayYMinimum=-2.7903298017751648  ActiveDisplayYMaximum=-1.7770998587100291  DataLoggingVariableName=ScopeData10
  "Sinusoidal Measurement (PLL, Three-Phase)" : eeSinusoidalMeasurementV2/Sinusoidal Measurement (PLL, Three-Phase)  InputFilter=on  InputNormalization=off  Kp_LF=40  Ki_LF=1000  F0=frequency  Theta0=0  Ts=Ts
  Terminator : Terminator
  Terminator1 : Terminator
  mag : Outport
  freq : Outport  Port=2
  angle : Outport  Port=3
  Vd : Outport  Port=4
  Vq : Outport  Port=5
  Id1 : Outport  Port=6
  Iq1 : Outport  Port=7
  wires:
  Iabc/1 -> Park Transform1/1
  Demux1/3 -> Terminator1/1
  Demux1/2 -> Scope1/2, Iq1/1
  Demux1/1 -> Scope1/1, Id1/1
  Park Transform1/1 -> Demux1/1
  "Sinusoidal Measurement (PLL, Three-Phase)"/3 -> mag/1
  "Sinusoidal Measurement (PLL, Three-Phase)"/1 -> freq/1
  "Sinusoidal Measurement (PLL, Three-Phase)"/2 -> Park Transform/2, Park Transform1/2, angle/1
  Demux/2 -> Vq/1, Scope/2
  Demux/1 -> Vd/1, Scope/1
  Park Transform/1 -> Demux/1
  Vabc/1 -> "Sinusoidal Measurement (PLL, Three-Phase)"/1, Park Transform/1
  Demux/3 -> Terminator/1
